simulink model "sim_luenburger_rdelay"  (Simulink 8.4)
settings: Solver=ode23s  StartTime=0.0  StopTime=2*max(time)  FixedStep=0.0001  RelTol=1e-3
values from neighbouring files (symbols this model uses):
  CTRL = ctrl_d(i)    [step3_analyse_export.m]    (also in step4_simulation.m = ctrl_d(5))
  PLANT = model.chip    [step2_design_controller.m]    (also in step3_analyse_export.m = model.combo; step4_simulation.m = model.combo)
  RESET_TIME = REFERENCE_STEP_DURATION*(1 + length(CTRL.output))    [step4_simulation.m]
libraries: simulink x4
settings Model: Creator=yh3wong  LastModifiedBy=yh3wong
settings DataIOCC: SignalLoggingSaveFormat=Dataset
settings OptimizationCC: ExpressionDepthLimit=128
settings DebuggingCC: UnderspecifiedInitializationDetection=Simplified  MergeDetectMultiDrivingBlocksExec=error  FcnCallInpInsideContextMsg=EnableAllAsError  StateNameClashWarn=none
settings GRTTargetCC: CombineOutputUpdateFcns=on  GRTInterface=off

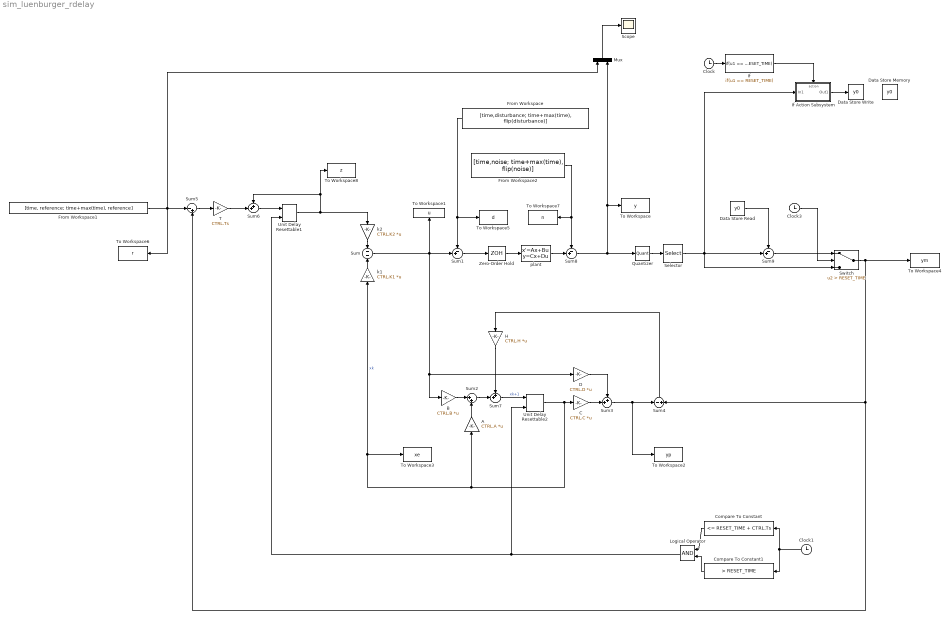
== system sim_luenburger_rdelay ==
  A : Gain  Gain=CTRL.A  Multiplication=Matrix(K*u)  SampleTime=CTRL.Ts
  B : Gain  Gain=CTRL.B  Multiplication=Matrix(K*u)  SampleTime=CTRL.Ts
  C : Gain  Gain=CTRL.C  Multiplication=Matrix(K*u)  SampleTime=CTRL.Ts
  Clock : Clock
  Clock1 : Clock
  Clock3 : Clock
  Compare To Constant : simulink/Logic and Bit Operations/Compare To Constant  relop=<=  const=RESET_TIME + CTRL.Ts  OutDataTypeStr=boolean
  Compare To Constant1 : simulink/Logic and Bit Operations/Compare To Constant  relop=>  const=RESET_TIME  OutDataTypeStr=boolean
  D : Gain  Gain=CTRL.D  Multiplication=Matrix(K*u)  SampleTime=CTRL.Ts
  Data Store Memory : DataStoreMemory  DataStoreName=y0  ReadBeforeWriteMsg=error  WriteAfterWriteMsg=error  WriteAfterReadMsg=error  InitialValue=zeros(size(CTRL.output))
  Data Store Read : DataStoreRead  DataStoreName=y0  SampleTime=CTRL.Ts
  Data Store Write : DataStoreWrite  DataStoreName=y0
  From Workspace : FromWorkspace  VariableName=[time,disturbance; time+max(time), flip(disturbance)]  SampleTime=CTRL.Ts  Interpolate=off  OutputAfterFinalValue=Holding final value
  From Workspace1 : FromWorkspace  VariableName=[time, reference; time+max(time), reference]  SampleTime=CTRL.Ts  Interpolate=off  OutputAfterFinalValue=Holding final value
  From Workspace2 : FromWorkspace  VariableName=[time,noise; time+max(time), flip(noise)]  SampleTime=CTRL.Ts  OutputAfterFinalValue=Holding final value
  H : Gain  Gain=CTRL.H  Multiplication=Matrix(K*u)  SampleTime=CTRL.Ts
  If : If  IfExpression=u1 == RESET_TIME  ShowElse=off
  If Action Subsystem : Subsystem  TreatAsAtomicUnit=on
  Logical Operator : Logic  AllPortsSameDT=off  OutDataTypeStr=boolean
  Mux : Mux  Inputs=2
  Quantizer : Quantizer  QuantizationInterval=DOUBT_SENSOR
  Scope : Scope
      settings: YMin=-150  YMax=200
  Selector : Selector  InputPortWidth=length(PLANT.output)  Indices=CTRL.channel_idx
  Sum : Sum  Inputs=-|-  SampleTime=CTRL.Ts
  Sum1 : Sum  Inputs=-+|  SampleTime=CTRL.Ts
  Sum2 : Sum  Inputs=|++  SampleTime=CTRL.Ts
  Sum3 : Sum  Inputs=++|  SampleTime=CTRL.Ts
  Sum4 : Sum  Inputs=-|+  SampleTime=CTRL.Ts
  Sum5 : Sum  Inputs=|-+  SampleTime=CTRL.Ts
  Sum6 : Sum  Inputs=++|  SampleTime=CTRL.Ts
  Sum7 : Sum  Inputs=++|  SampleTime=CTRL.Ts
  Sum8 : Sum  Inputs=-+|
  Sum9 : Sum  Inputs=-+|  SampleTime=CTRL.Ts
  Switch : Switch  Criteria=u2 > Threshold  Threshold=RESET_TIME  SampleTime=CTRL.Ts
  T : Gain  Gain=CTRL.Ts  SampleTime=CTRL.Ts
  To Workspace : ToWorkspace  VariableName=y  SaveFormat=Structure With Time  SampleTime=-1
  To Workspace1 : ToWorkspace  VariableName=u  SaveFormat=Structure With Time  SampleTime=CTRL.Ts
  To Workspace2 : ToWorkspace  VariableName=yp  SaveFormat=Structure With Time  SampleTime=CTRL.Ts
  To Workspace3 : ToWorkspace  VariableName=xe  SaveFormat=Structure With Time  SampleTime=CTRL.Ts
  To Workspace4 : ToWorkspace  VariableName=ym  SaveFormat=Structure With Time  SampleTime=-1
  To Workspace5 : ToWorkspace  VariableName=d  SaveFormat=Structure With Time  SampleTime=CTRL.Ts
  To Workspace6 : ToWorkspace  VariableName=r  SaveFormat=Structure With Time  SampleTime=CTRL.Ts
  To Workspace7 : ToWorkspace  VariableName=n  SaveFormat=Structure With Time  SampleTime=CTRL.Ts
  To Workspace8 : ToWorkspace  VariableName=z  SaveFormat=Structure With Time  SampleTime=CTRL.Ts
  Unit Delay Resettable1 : simulink/Additional Math & Discrete/Additional Discrete/Unit Delay Resettable  vinit=zeros(size(CTRL.output))  tsamp=CTRL.Ts
  Unit Delay Resettable2 : simulink/Additional Math & Discrete/Additional Discrete/Unit Delay Resettable  vinit=zeros(size(CTRL.state))  tsamp=CTRL.Ts
  Zero-Order Hold : ZeroOrderHold  SampleTime=CTRL.Ts
  "k1 " : Gain  Gain=CTRL.K1  Multiplication=Matrix(K*u)  SampleTime=CTRL.Ts
  k2 : Gain  Gain=CTRL.K2  Multiplication=Matrix(K*u)  SampleTime=CTRL.Ts
  plant : StateSpace  A=PLANT.Ac  B=PLANT.Bc  C=PLANT.Cc  D=PLANT.Dc  X0=0
  wires:
  k2/1 -> Sum/1
  "k1 "/1 -> Sum/2
  Zero-Order Hold/1 -> plant/1
  From Workspace/1 -> Sum1/1, To Workspace5/1
  Sum1/1 -> Zero-Order Hold/1
  Sum3/1 -> Sum4/1, To Workspace2/1
  Sum5/1 -> T/1
  plant/1 -> Sum8/2
  From Workspace1/1 -> Sum5/1, To Workspace6/1, Mux/1
  Mux/1 -> Scope/1
  D/1 -> Sum3/1
  C/1 -> Sum3/2
  If/1 -> If Action Subsystem/Action
  If Action Subsystem/1(Out1) -> Data Store Write/1
  Sum9/1 -> Switch/1
  Data Store Read/1 -> Sum9/1
  Clock/1 -> If/1
  Clock3/1 -> Switch/2
  Selector/1 -> If Action Subsystem/1(In1), Switch/3, Sum9/2
  From Workspace2/1 -> To Workspace7/1, Sum8/1
  Quantizer/1 -> Selector/1
  Sum8/1 -> Quantizer/1, To Workspace/1, Mux/2
  Clock1/1 -> Compare To Constant/1, Compare To Constant1/1
  Compare To Constant/1 -> Logical Operator/1
  Compare To Constant1/1 -> Logical Operator/2
  A/1 -> Sum2/2
  B/1 -> Sum2/1
  H/1 -> Sum7/1
  Sum4/1 -> H/1
  Switch/1 -> To Workspace4/1, Sum4/2, Sum5/2
  Sum/1 -> B/1, D/1, To Workspace1/1, Sum1/2
  Sum2/1 -> Sum7/2
  Sum7/1 -> Unit Delay Resettable2/1  "xk+1"
  Logical Operator/1 -> Unit Delay Resettable1/2, Unit Delay Resettable2/2
  Unit Delay Resettable2/1 -> C/1, To Workspace3/1, "k1 "/1, A/1  "xk"
  Sum6/1 -> Unit Delay Resettable1/1
  Unit Delay Resettable1/1 -> Sum6/1, To Workspace8/1, k2/1
  T/1 -> Sum6/2

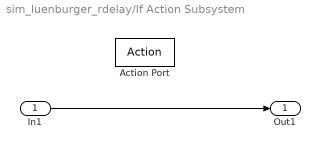
== system sim_luenburger_rdelay/If Action Subsystem ==
  In1 : Inport
  Action Port : ActionPort  ActionType=then
  Out1 : Outport
  wires:
  In1/1 -> Out1/1
